simulink model "Data_Net_8_31_31_2"  (R2026a)
settings: Solver=FixedStepAuto
undefined symbols (not defined in the file or in its folder): net_trained
libraries: dlconvfclib x3, dlactivationlib x3, dlutilitylib x1
settings Model: Creator=emil  LastModifiedBy=emil
settings RTWCC: SystemTargetFile=ert.tlc  Description=Embedded Coder
settings ERTTargetCC: GenerateSampleERTMain=on

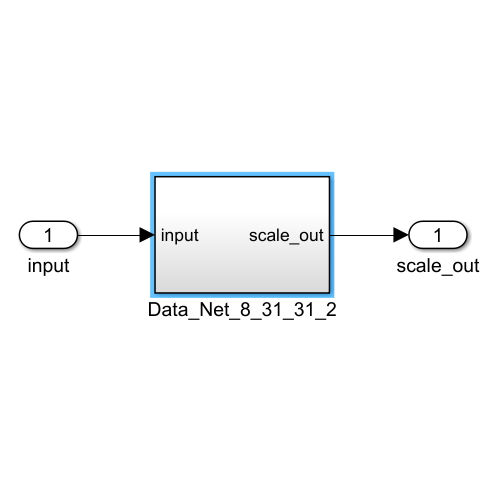
[thumbnail: Simulink's stored preview of the top-level diagram]
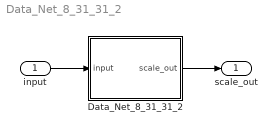
== system Data_Net_8_31_31_2 ==
  input : Inport  PortDimensions=[8]
  Data_Net_8_31_31_2 : Subsystem
  scale_out : Outport
  wires:
  input/1 -> Data_Net_8_31_31_2/1(input)
  Data_Net_8_31_31_2/1(scale_out) -> scale_out/1

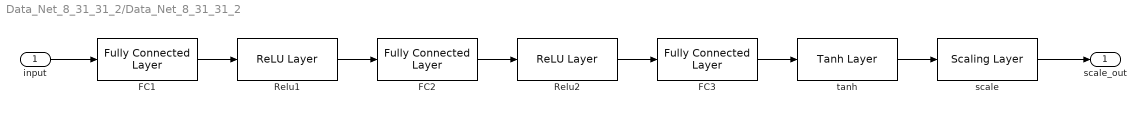
== system Data_Net_8_31_31_2/Data_Net_8_31_31_2 ==
  input : Inport  PortDimensions=[8]
  FC1 : dlconvfclib/Fully Connected Layer  Layer=net_trained.Layers(2)  OutMin=[]  OutMax=[]  WeightsDataTypeStr=Inherit: Inherit via back propagation  WeightsMin=[]  WeightsMax=[]  BiasDataTypeStr=Inherit: Inherit via back propagation  BiasMin=[]  BiasMax=[]  AccumMin=[]  AccumMax=[]  InternalRndMeth=Floor  InternalSaturateOnIntegerOverflow=off  SampleTime=-1
      settings: DataFormat=C
  FC2 : dlconvfclib/Fully Connected Layer  Layer=net_trained.Layers(4)  OutMin=[]  OutMax=[]  WeightsDataTypeStr=Inherit: Inherit via back propagation  WeightsMin=[]  WeightsMax=[]  BiasDataTypeStr=Inherit: Inherit via back propagation  BiasMin=[]  BiasMax=[]  AccumMin=[]  AccumMax=[]  InternalRndMeth=Floor  InternalSaturateOnIntegerOverflow=off  SampleTime=-1
      settings: DataFormat=C
  FC3 : dlconvfclib/Fully Connected Layer  Layer=net_trained.Layers(6)  OutMin=[]  OutMax=[]  WeightsDataTypeStr=Inherit: Inherit via back propagation  WeightsMin=[]  WeightsMax=[]  BiasDataTypeStr=Inherit: Inherit via back propagation  BiasMin=[]  BiasMax=[]  AccumMin=[]  AccumMax=[]  InternalRndMeth=Floor  InternalSaturateOnIntegerOverflow=off  SampleTime=-1
      settings: DataFormat=C
  Relu1 : dlactivationlib/ReLU Layer  OutMin=[]  OutMax=[]  SampleTime=-1
  Relu2 : dlactivationlib/ReLU Layer  OutMin=[]  OutMax=[]  SampleTime=-1
  scale : dlutilitylib/Scaling Layer  Scale=net_trained.Layers(8).Scale  OutMin=[]  OutMax=[]  ScaleDataTypeStr=Inherit: Inherit via back propagation  ScaleMin=[]  ScaleMax=[]  OffsetDataTypeStr=Inherit: Inherit via back propagation  OffsetMin=[]  OffsetMax=[]  AccumMin=[]  AccumMax=[]  InternalRndMeth=Floor  InternalSaturateOnIntegerOverflow=off  SampleTime=-1  Offset=net_trained.Layers(8).Offset
      settings: DataFormat=C
  tanh : dlactivationlib/Tanh Layer  ApproximationMethod=None  OutMin=[]  OutMax=[]  SampleTime=-1
  scale_out : Outport
  wires:
  FC3/1 -> tanh/1
  FC2/1 -> Relu2/1
  tanh/1 -> scale/1
  input/1 -> FC1/1
  Relu2/1 -> FC3/1
  FC1/1 -> Relu1/1
  scale/1 -> scale_out/1
  Relu1/1 -> FC2/1
